simulink model "dynamiczny_dyskretny_model_zlinearyzowany"  (R2021a)
settings: Solver=VariableStepAuto  StartTime=0.0  StopTime=10.0  RelTol=1e-3
values from neighbouring files (symbols this model uses):
  T = 0.5    [z3_czas_probkowania_T.m]    (also in z9_czas_probkowania_T_wartosc_ud.m = 1)
  ud = [-1:0.1:1]    [z11_transmitacja_wykres.m]    (also in z6_zlinearyzowana_charakterystyka_statyczna.m = -1; z9_czas_probkowania_T_wartosc_ud.m = 0.5)
settings Model: Creator=48604  LastModifiedBy=48604

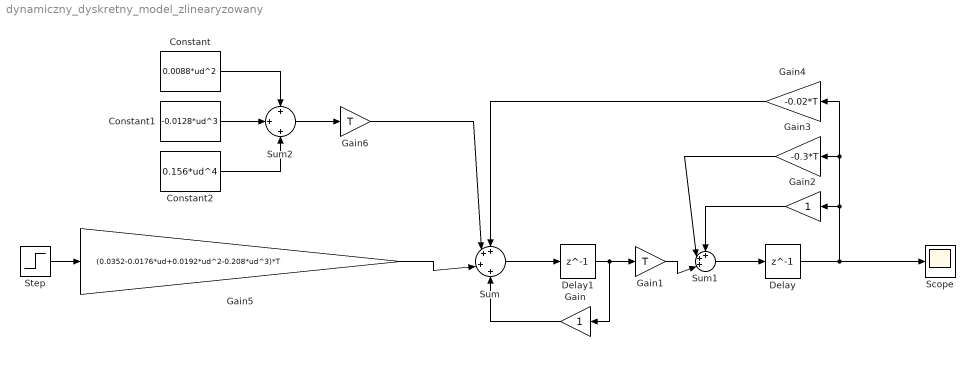
== system dynamiczny_dyskretny_model_zlinearyzowany ==
  Constant : Constant  Value=0.0088*ud^2
  Constant1 : Constant  Value=-0.0128*ud^3
  Constant2 : Constant  Value=0.156*ud^4
  Delay : Delay  DelayLength=1  InitialCondition=0
  Delay1 : Delay  DelayLength=1  InitialCondition=0
  Gain : Gain
  Gain1 : Gain  Gain=T
  Gain2 : Gain
  Gain3 : Gain  Gain=-0.3*T
  Gain4 : Gain  Gain=-0.02*T
  Gain5 : Gain  Gain=(0.0352-0.0176*ud+0.0192*ud^2-0.208*ud^3)*T
  Gain6 : Gain  Gain=T
  Scope : Scope
  Step : Step  SampleTime=0
  Sum : Sum  Inputs=++|+|+
  Sum1 : Sum  Inputs=+++|
  Sum2 : Sum  Inputs=+|+|+
  wires:
  Delay1/1 -> Gain/1, Gain1/1
  Gain1/1 -> Sum1/3
  Delay/1 -> Gain4/1, Gain3/1, Gain2/1, Scope/1
  Sum1/1 -> Delay/1
  Gain3/1 -> Sum1/2
  Gain2/1 -> Sum1/1
  Sum/1 -> Delay1/1
  Step/1 -> Gain5/1
  Constant/1 -> Sum2/1
  Constant1/1 -> Sum2/2
  Constant2/1 -> Sum2/3
  Sum2/1 -> Gain6/1
  Gain/1 -> Sum/4
  Gain5/1 -> Sum/3
  Gain6/1 -> Sum/2
  Gain4/1 -> Sum/1
